simulink model "kestane"  (R2021b)
settings: Solver=VariableStepAuto  StartTime=0.0  StopTime=70  RelTol=1e-3
values from neighbouring files (symbols this model uses):
  g = vpa(simplify(g),4)    [dynamic.m]
  k = 4e-2    (= 0.04)    [trajectory_computation.m]
undefined symbols (not defined in the file or in its folder): sigbuilder_block, X, Y, Z
libraries: sm_lib x139, nesl_utility x13, Contact_Forces_Lib x1
(part 5 of 5)

== system kestane/Kestane/Top spike6 ==
  Brick Solid5 : sm_lib/Body Elements/Brick Solid  GraphicAmbientColor=[0.15 0.15 0.15 1.0]  BasedOnType=Density  BrickDimensions=[k 0.005 0.005]  BrickDimensionUnits=m  CenterOfMass=[0 0 0]  CenterOfMassUnits=cm  GraphicDiffuseColor=[0.5 0.5 0.5]  Density=100  DensityUnits=g/cm^3  DoExposeReferenceFrame=on  GraphicEmissiveColor=[0.0 0.0 0.0 1.0]  ExportEntireGeometry=on  SerializedFrames=<Frames><Frame><Id>Frame1</Id><Value><Name>F1</Name><Origin><Source>GeometricFeature</Source><FeatureName>+x surface</FeatureName></Origin><PrimaryAxis><DefinedDirection>+Z</DefinedDirection><Source>GeometricFeature</Source><SourceDirection>+Z</SourceDirection><FeatureName>+x surface</FeatureName></PrimaryAxis><SecondaryAxis><DefinedDirection>-Y</DefinedDirection><Source>GeometricFeature</Source><SourceDirection>+X</SourceDirection><FeatureName>+x -y curve</FeatureName></SecondaryAxis></Value></Frame><Frame><Id>Frame2</Id><Value><Name>F2</Name><Origin><Source>GeometricFeature</Source><FeatureName>-x surface</FeatureName></Origin><PrimaryAxis><DefinedDirection>-Z</DefinedDirection><Source>GeometricFeature</Source><SourceDirection>+Z</SourceDirection><FeatureName>-x surface</FeatureName></PrimaryAxis><SecondaryAxis><DefinedDirection>-X</DefinedDirection><Source>GeometricFeature</Source><SourceDirection>+X</SourceDirection><FeatureName>+z -x curve</FeatureName></SecondaryAxis></Value></Frame></Frames>  MarkerShape=Sphere  MarkerSize=10  GraphicType=FromGeometry  InertiaType=Custom  Mass=10  MassUnits=g  MomentsOfInertia=[1e-15 1e-15 1e-15]  MomentsOfInertiaUnits=g*cm^2  GraphicOpacity=1.0  ProductsOfInertia=[0 0 0]  ProductsOfInertiaUnits=kg*m^2  GraphicShininess=75  GraphicSpecularColor=[0.5 0.5 0.5 1.0]  GraphicVisPropType=SimpleVisualProperties
  Cylindrical Solid : sm_lib/Body Elements/Cylindrical Solid  GraphicAmbientColor=[0.15 0.15 0.15 1.0]  BasedOnType=Density  CenterOfMass=[0 0 0]  CenterOfMassUnits=cm  GraphicDiffuseColor=[0.5 0.5 0.5]  CylinderLength=r  CylinderLengthUnits=m  CylinderRadius=0.25  CylinderRadiusUnits=cm  Density=100  DensityUnits=g/cm^3  DoExposeReferenceFrame=on  GraphicEmissiveColor=[0.0 0.0 0.0 1.0]  ExportEntireGeometry=on  SerializedFrames=<Frames><Frame><Id>Frame1</Id><Value><Name>F1</Name><Origin><Source>GeometricFeature</Source><FeatureName>top surface</FeatureName></Origin><PrimaryAxis><DefinedDirection>+Z</DefinedDirection><Source>ReferenceFrame</Source><SourceDirection>+Z</SourceDirection><FeatureName></FeatureName></PrimaryAxis><SecondaryAxis><DefinedDirection>+X</DefinedDirection><Source>ReferenceFrame</Source><SourceDirection>+X</SourceDirection><FeatureName></FeatureName></SecondaryAxis></Value></Frame><Frame><Id>Frame2</Id><Value><Name>F2</Name><Origin><Source>GeometricFeature</Source><FeatureName>top surface</FeatureName></Origin><PrimaryAxis><DefinedDirection>+Z</DefinedDirection><Source>ReferenceFrame</Source><SourceDirection>+Z</SourceDirection><FeatureName></FeatureName></PrimaryAxis><SecondaryAxis><DefinedDirection>+X</DefinedDirection><Source>ReferenceFrame</Source><SourceDirection>+X</SourceDirection><FeatureName></FeatureName></SecondaryAxis></Value></Frame></Frames>  MarkerShape=Sphere  MarkerSize=10  GraphicType=FromGeometry  InertiaType=Custom  Mass=50  MassUnits=g  MomentsOfInertia=[1e-15 1e-15 1e-15]  MomentsOfInertiaUnits=g*cm^2  GraphicOpacity=1.0  ProductsOfInertia=[0 0 0]  ProductsOfInertiaUnits=kg*m^2  GraphicShininess=75  GraphicSpecularColor=[0.5 0.5 0.5 1.0]  GraphicVisPropType=SimpleVisualProperties
  Prismatic Joint5 : sm_lib/Joints/Prismatic Joint  JointMode=Normal  SenseConstraintForce=off  SenseConstraintForceX=off  SenseConstraintForceY=off  SenseConstraintForceZ=off  SenseConstraintTorque=off  SenseConstraintTorqueX=off  SenseConstraintTorqueY=off  SenseConstraintTorqueZ=off  SenseTotalForce=off  SenseTotalForceX=off  SenseTotalForceY=off  SenseTotalForceZ=off  SenseTotalTorque=off  SenseTotalTorqueX=off  SenseTotalTorqueY=off  SenseTotalTorqueZ=off  CompositeWrenchDir=FollowerOnBase  CompositeWrenchFrame=BaseFrame  EquilibriumPosition=0  EquilibriumPositionUnits=cm  SpringStiffness=10  SpringStiffnessUnits=N/m  DampingCoefficient=10  DampingCoefficientUnits=N/(m/s)  TorqueActuationMode=NoTorque  MotionActuationMode=ComputedMotion  SensePosition=off  SenseVelocity=off  SenseAcceleration=off  SenseTorqueForce=off  SenseLowerLimitTorqueForce=off  SenseUpperLimitTorqueForce=off  LowerLimitSpecify=on  LowerLimitBound=1  LowerLimitBoundUnits=cm  LowerLimitStiffness=1e3  LowerLimitStiffnessUnits=N/m  LowerLimitDamping=1e3  LowerLimitDampingUnits=N/(m/s)  LowerLimitTransitionRegionWidth=1e-4  LowerLimitTransitionRegionWidthUnits=m  UpperLimitSpecify=on  UpperLimitBound=2  UpperLimitBoundUnits=cm  UpperLimitStiffness=1e4  UpperLimitStiffnessUnits=N/m  UpperLimitDamping=1e4  UpperLimitDampingUnits=N/(m/s)  UpperLimitTransitionRegionWidth=1e-4  UpperLimitTransitionRegionWidthUnits=m  PositionTargetSpecify=on  PositionTargetPriority=High  PositionTargetValue=1.5  PositionTargetValueUnits=cm  VelocityTargetSpecify=on  VelocityTargetPriority=High  VelocityTargetValue=0  VelocityTargetValueUnits=m/s
  Revolute Joint11 : sm_lib/Joints/Revolute Joint  JointMode=Normal  SenseConstraintForce=off  SenseConstraintForceX=off  SenseConstraintForceY=off  SenseConstraintForceZ=off  SenseConstraintTorque=off  SenseConstraintTorqueX=off  SenseConstraintTorqueY=off  SenseConstraintTorqueZ=off  SenseTotalForce=off  SenseTotalForceX=off  SenseTotalForceY=off  SenseTotalForceZ=off  SenseTotalTorque=off  SenseTotalTorqueX=off  SenseTotalTorqueY=off  SenseTotalTorqueZ=off  CompositeWrenchDir=FollowerOnBase  CompositeWrenchFrame=BaseFrame  EquilibriumPosition=0  EquilibriumPositionUnits=deg  SpringStiffness=0  SpringStiffnessUnits=N*m/deg  DampingCoefficient=1e10  DampingCoefficientUnits=N*m/(deg/s)  TorqueActuationMode=NoTorque  MotionActuationMode=ComputedMotion  SensePosition=off  SenseVelocity=off  SenseAcceleration=off  SenseTorqueForce=off  SenseLowerLimitTorqueForce=off  SenseUpperLimitTorqueForce=off  LowerLimitSpecify=on  LowerLimitBound=82  LowerLimitBoundUnits=deg  LowerLimitStiffness=0  LowerLimitStiffnessUnits=N*m/deg  LowerLimitDamping=1e10  LowerLimitDampingUnits=N*m/(deg/s)  LowerLimitTransitionRegionWidth=0.1  LowerLimitTransitionRegionWidthUnits=deg  UpperLimitSpecify=on  UpperLimitBound=98  UpperLimitBoundUnits=deg  UpperLimitStiffness=0  UpperLimitStiffnessUnits=N*m/deg  UpperLimitDamping=1e10  UpperLimitDampingUnits=N*m/(deg/s)  UpperLimitTransitionRegionWidth=0.1  UpperLimitTransitionRegionWidthUnits=deg  PositionTargetSpecify=on  PositionTargetPriority=High  PositionTargetValue=90  PositionTargetValueUnits=deg  VelocityTargetSpecify=off  VelocityTargetPriority=High  VelocityTargetValue=0  VelocityTargetValueUnits=deg/s
  Revolute Joint5 : sm_lib/Joints/Revolute Joint  JointMode=Normal  SenseConstraintForce=off  SenseConstraintForceX=off  SenseConstraintForceY=off  SenseConstraintForceZ=off  SenseConstraintTorque=off  SenseConstraintTorqueX=off  SenseConstraintTorqueY=off  SenseConstraintTorqueZ=off  SenseTotalForce=off  SenseTotalForceX=off  SenseTotalForceY=off  SenseTotalForceZ=off  SenseTotalTorque=off  SenseTotalTorqueX=off  SenseTotalTorqueY=off  SenseTotalTorqueZ=off  CompositeWrenchDir=FollowerOnBase  CompositeWrenchFrame=BaseFrame  EquilibriumPosition=-30  EquilibriumPositionUnits=deg  SpringStiffness=1  SpringStiffnessUnits=N*m/deg  DampingCoefficient=1  DampingCoefficientUnits=N*m/(deg/s)  TorqueActuationMode=NoTorque  MotionActuationMode=ComputedMotion  SensePosition=off  SenseVelocity=off  SenseAcceleration=off  SenseTorqueForce=off  SenseLowerLimitTorqueForce=off  SenseUpperLimitTorqueForce=off  LowerLimitSpecify=on  LowerLimitBound=-31  LowerLimitBoundUnits=deg  LowerLimitStiffness=1e4  LowerLimitStiffnessUnits=N*m/deg  LowerLimitDamping=10  LowerLimitDampingUnits=N*m/(deg/s)  LowerLimitTransitionRegionWidth=0.1  LowerLimitTransitionRegionWidthUnits=deg  UpperLimitSpecify=on  UpperLimitBound=-29  UpperLimitBoundUnits=deg  UpperLimitStiffness=1e4  UpperLimitStiffnessUnits=N*m/deg  UpperLimitDamping=10  UpperLimitDampingUnits=N*m/(deg/s)  UpperLimitTransitionRegionWidth=0.1  UpperLimitTransitionRegionWidthUnits=deg  PositionTargetSpecify=on  PositionTargetPriority=High  PositionTargetValue=-30  PositionTargetValueUnits=deg  VelocityTargetSpecify=on  VelocityTargetPriority=High  VelocityTargetValue=0  VelocityTargetValueUnits=deg/s
  Rigid Transform10 : sm_lib/Frames and Transforms/Rigid Transform  TranslationMethod=None  TranslationStandardOffset=0  TranslationLengthUnit=m  TranslationStandardAxis=+Z  TranslationCartesianOffset=[0 0 0]  TranslationROffset=0  TranslationROffsetUnits=m  TranslationZOffset=0  TranslationZOffsetUnits=m  TranslationThetaOffset=0  TranslationThetaOffsetUnits=deg  RotationMethod=StandardAxis  RotationAngleUnits=deg  RotationStandardAxis=+X  RotationAngle=90.0  RotationArbitraryAxis=[0 0 1]  FollAlignAxisA=+X  BaseAlignAxisA=+Y  FollAlignAxisB=+Y  BaseAlignAxisB=+Z  RotationSequenceAxes=FollowerAxes  RotationSequence=XYX  RotationSequenceAngles=[0 0 0]  RotationSequenceAnglesUnits=deg  RotationMatrix=[1 0 0; 0 1 0; 0 0 1]
  Rigid Transform16 : sm_lib/Frames and Transforms/Rigid Transform  TranslationMethod=StandardAxis  TranslationStandardOffset=0.5  TranslationLengthUnit=cm  TranslationStandardAxis=+Z  TranslationCartesianOffset=[0 0 0]  TranslationROffset=0  TranslationROffsetUnits=m  TranslationZOffset=0  TranslationZOffsetUnits=m  TranslationThetaOffset=0  TranslationThetaOffsetUnits=deg  RotationMethod=None  RotationAngleUnits=deg  RotationStandardAxis=+Z  RotationAngle=0.0  RotationArbitraryAxis=[0 0 1]  FollAlignAxisA=+X  BaseAlignAxisA=+Y  FollAlignAxisB=+Y  BaseAlignAxisB=+Z  RotationSequenceAxes=FollowerAxes  RotationSequence=XYX  RotationSequenceAngles=[0 0 0]  RotationSequenceAnglesUnits=deg  RotationMatrix=[1 0 0; 0 1 0; 0 0 1]
  Rigid Transform22 : sm_lib/Frames and Transforms/Rigid Transform  TranslationMethod=None  TranslationStandardOffset=0  TranslationLengthUnit=m  TranslationStandardAxis=+Z  TranslationCartesianOffset=[0 0 0]  TranslationROffset=0  TranslationROffsetUnits=m  TranslationZOffset=0  TranslationZOffsetUnits=m  TranslationThetaOffset=0  TranslationThetaOffsetUnits=deg  RotationMethod=StandardAxis  RotationAngleUnits=deg  RotationStandardAxis=+X  RotationAngle=90.0  RotationArbitraryAxis=[0 0 1]  FollAlignAxisA=+X  BaseAlignAxisA=+Y  FollAlignAxisB=+Y  BaseAlignAxisB=+Z  RotationSequenceAxes=FollowerAxes  RotationSequence=XYX  RotationSequenceAngles=[0 0 0]  RotationSequenceAnglesUnits=deg  RotationMatrix=[1 0 0; 0 1 0; 0 0 1]
  Rigid Transform5 : sm_lib/Frames and Transforms/Rigid Transform  TranslationMethod=Cartesian  TranslationStandardOffset=0  TranslationLengthUnit=cm  TranslationStandardAxis=+Z  TranslationCartesianOffset=[-1.5*sqrt(3) 0 +1.5]  TranslationROffset=0  TranslationROffsetUnits=m  TranslationZOffset=0  TranslationZOffsetUnits=m  TranslationThetaOffset=0  TranslationThetaOffsetUnits=deg  RotationMethod=RotationMatrix  RotationAngleUnits=deg  RotationStandardAxis=+Z  RotationAngle=0.0  RotationArbitraryAxis=[0 0 1]  FollAlignAxisA=+X  BaseAlignAxisA=+Y  FollAlignAxisB=+Y  BaseAlignAxisB=+Z  RotationSequenceAxes=FollowerAxes  RotationSequence=XYX  RotationSequenceAngles=[0 0 0]  RotationSequenceAnglesUnits=deg  RotationMatrix=[-1 0 0;0 0 -1; 0 -1 0]
  Spatial Contact Force5 : sm_lib/Forces and Torques/Spatial Contact Force  CoefficientOfDynamicFriction=0.5  CoefficientOfStaticFriction=0.7  SenseContactBaseRotation=off  SenseContactBaseTranslation=off  NormalDamping=10  NormalDampingUnits=N/(m/s)  SenseContactFollowerRotation=off  SenseContactFollowerTranslation=off  SenseContactSignal=off  NormalStiffness=1e6  NormalStiffnessUnits=N/m  FrictionalCriticalVelocity=1e-3  FrictionalCriticalVelocityUnits=m/s  ZeroCrossDetectContactStartAndEnd=off  FrictionType=SmoothStickSlip  SenseFrictionalForceMagnitude=off  SenseNormalForceMagnitude=off  NormalForceType=SmoothSpringDamper  SenseNormalVelocity=off  SenseSeparationDistance=off  SenseTangentialVelocity=off  SenseTangentialVelocityMagnitude=off  NormalTransitionRegionWidth=1e-4  NormalTransitionRegionWidthUnits=m
  Spherical Solid5 : sm_lib/Body Elements/Spherical Solid  GraphicAmbientColor=[0.15 0.15 0.15 1.0]  BasedOnType=Mass  CenterOfMass=[0 0 0]  CenterOfMassUnits=m  GraphicDiffuseColor=[0.5 0.5 0.5]  Density=1000  DensityUnits=kg/m^3  DoExposeReferenceFrame=on  GraphicEmissiveColor=[0.0 0.0 0.0 1.0]  ExportEntireGeometry=on  SerializedExposedGeometries=<ExposedGeometries><ExposedGeometry><RawGeometryId>entire</RawGeometryId><ExposedGeometryId>G</ExposedGeometryId></ExposedGeometry></ExposedGeometries>  SerializedFrames=<Frames/>  MarkerShape=Sphere  MarkerSize=10  GraphicType=FromGeometry  InertiaType=CalculateFromGeometry  Mass=5  MassUnits=g  MomentsOfInertia=[1 1 1]  MomentsOfInertiaUnits=kg*m^2  GraphicOpacity=1.0  ProductsOfInertia=[0 0 0]  ProductsOfInertiaUnits=kg*m^2  GraphicShininess=75  GraphicSpecularColor=[0.5 0.5 0.5 1.0]  SphereRadius=0.5  SphereRadiusUnits=cm  GraphicVisPropType=SimpleVisualProperties
  Conn1 : PMIOPort  Side=Left
  Conn5 : PMIOPort  Port=2  Side=Left
  connections:
  Prismatic Joint5/LConn1 -- Brick Solid5/LConn1
  Rigid Transform10/RConn1 -- Revolute Joint11/LConn1
  Rigid Transform5/RConn1 -- Revolute Joint5/LConn1
  Rigid Transform10/LConn1 -- Revolute Joint5/RConn1
  Spherical Solid5/LConn1 -- Spatial Contact Force5/RConn1
  Rigid Transform16/RConn1 -- Spherical Solid5/RConn1
  Prismatic Joint5/RConn1 -- Cylindrical Solid/LConn2
  Rigid Transform22/LConn1 -- Revolute Joint11/RConn1
  Cylindrical Solid/LConn1 -- Rigid Transform16/LConn1
  Rigid Transform22/RConn1 -- Brick Solid5/LConn2
  Spatial Contact Force5/LConn1 -- Conn5/RConn1
  Conn1/RConn1 -- Rigid Transform5/LConn1

== system kestane/Kestane/Spike 1/Signal Builder ==
  Demux : Demux  Tag=STV Demux  Outputs=3
      settings: DisplayOption=none
  FromWs : FromWorkspace  Tag=STV FromWs  VariableName=tuvar
      SigBuilderData=|
      | common.afterFinalStr = 'Extrapolate'
      | common.sampleTime = 0
      | dataSet.timeRange = [0 70]
      | dataSet.name = 'Group 1'
      | sbobj.Groups.Name = 'Group 1'
      | sbobj.Groups.Signals(1).Name = 'theta1v'
      | sbobj.Groups.Signals(1).XData = [0 1 1.02004008016 1.04008016032 1.06012024048 1.08016032064 1.1002004008 1.12024048096 1.14028056112 1.16032064128 1.18036072144 1.2004008016 ... (5001 elements, 1x5001)]
      | sbobj.Groups.Signals(1).YData = [-1.33121558998e-05 -1.33121558998e-05 -5.28852062004e-05 -0.000170609462846 -0.000364414136278 -0.00063215837707 -0.000971723764753 -0.00138101533953 -0.00185796251377 -0.00240051986857 -0.00300666784074 -0.00367441330488 ... (5001 elements, 1x5001)]
      | sbobj.Groups.Signals(2).Name = 'theta2v'
      | sbobj.Groups.Signals(2).XData = [0 1 1.02004008016 1.04008016032 1.06012024048 1.08016032064 1.1002004008 1.12024048096 1.14028056112 1.16032064128 1.18036072144 1.2004008016 ... (5002 elements, 1x5002)]
      | sbobj.Groups.Signals(2).YData = [9.17654507937e-07 9.17654507937e-07 3.66528587481e-06 1.18935666149e-05 2.5572133272e-05 4.46698421197e-05 6.91564068234e-05 9.90026718162e-05 0.000134180855199 0.000174664762492 0.000220429972497 0.000271453996453 ... (5002 elements, 1x5002)]
      | sbobj.Groups.Signals(3).Name = 'd3v'
      | sbobj.Groups.Signals(3).XData = [0 1 1.02004008016 1.04008016032 1.06012024048 1.08016032064 1.1002004008 1.12024048096 1.14028056112 1.16032064128 1.18036072144 1.2004008016 ... (5002 elements, 1x5002)]
      | sbobj.Groups.Signals(3).YData = [-2.27265007507e-07 -2.27265007507e-07 -9.03146913159e-07 -2.91455572836e-06 -6.22754426326e-06 -1.08066210217e-05 -1.66160796084e-05 -2.36198607756e-05 -3.17814304776e-05 -4.10636731864e-05 -5.14287997626e-05 -6.28382692144e-05 ... (5002 elements, 1x5002)]
      | sbobj.Groups.TimeRange = [0 70]
  theta1v : Outport  Tag=STV Outport
  theta2v : Outport  Tag=STV Outport  Port=2
  d3v : Outport  Tag=STV Outport  Port=3
  wires:
  Demux/1 -> theta1v/1
  FromWs/1 -> Demux/1
  Demux/2 -> theta2v/1
  Demux/3 -> d3v/1

== system kestane/Kestane/Spike 4/Spike 1 Driver ==
  Demux : Demux  Tag=STV Demux  Outputs=3
      settings: DisplayOption=none
  FromWs : FromWorkspace  Tag=STV FromWs  VariableName=tuvar
      SigBuilderData=|
      | common.afterFinalStr = 'Extrapolate'
      | common.sampleTime = 0
      | dataSet.timeRange = [0 70]
      | dataSet.name = 'Group 1'
      | sbobj.Groups.Name = 'Group 1'
      | sbobj.Groups.Signals(1).Name = 'theta1'
      | sbobj.Groups.Signals(1).XData = [0 1 1.02004008016 1.04008016032 1.06012024048 1.08016032064 1.1002004008 1.12024048096 1.14028056112 1.16032064128 1.18036072144 1.2004008016 ... (4997 elements, 1x4997)]
      | sbobj.Groups.Signals(1).YData = [0.523598775598 0.523598775598 0.523598509355 0.52359666019 0.523591684977 0.523582083625 0.523566398642 0.523543214674 0.523511158028 0.523468896173 0.523415137233 0.52334862946 ... (4997 elements, 1x4997)]
      | sbobj.Groups.Signals(2).Name = 'd3'
      | sbobj.Groups.Signals(2).XData = [0 1 1.02004008016 1.04008016032 1.06012024048 1.08016032064 1.1002004008 1.12024048096 1.14028056112 1.16032064128 1.18036072144 1.2004008016 ... (4998 elements, 1x4998)]
      | sbobj.Groups.Signals(2).YData = [0.0120221607105 0.0120221607105 0.0120221561652 0.0120221245847 0.012022039583 0.0120218754829 0.0120216073182 0.0120212108397 0.0120206625237 0.0120199395825 0.0120190199768 0.0120178824305 ... (4998 elements, 1x4998)]
      | sbobj.Groups.Signals(3).Name = 'theta2'
      | sbobj.Groups.Signals(3).XData = [0 1 1.02004008016 1.04008016032 1.06012024048 1.08016032064 1.1002004008 1.12024048096 1.14028056112 1.16032064128 1.18036072144 1.2004008016 ... (4998 elements, 1x4998)]
      | sbobj.Groups.Signals(3).YData = [1.7345311581 1.7345311581 1.73453113975 1.73453101149 1.73453066401 1.73452998861 1.73452887721 1.73452722235 1.73452491711 1.73452185512 1.73451793052 1.73451303792 ... (4998 elements, 1x4998)]
      | sbobj.Groups.TimeRange = [0 70]
  theta1 : Outport  Tag=STV Outport
  d3 : Outport  Tag=STV Outport  Port=2
  theta2 : Outport  Tag=STV Outport  Port=3
  wires:
  FromWs/1 -> Demux/1
  Demux/1 -> theta1/1
  Demux/2 -> d3/1
  Demux/3 -> theta2/1

== matlab function kestane/Kestane/Spike 1/MATLAB Function ==
  data: theta1 input; t1 output; theta2 input; d3 input; theta1v input; theta2v input; d3v input; theta1vd input; theta2vd input; d3vd input; theta1d input; theta2d input; d3d input; t2 output; t3 output
function [t1,t2,t3] = force_control(theta1,theta2,d3,theta1v,theta2v,d3v,theta1vd,theta2vd,d3vd,theta1d,theta2d,d3d)
x = (0.04+d3);
J = [-x*sin(theta1)*sin(theta2) x*cos(theta1)*cos(theta2) cos(theta1)*sin(theta2);
    x*cos(theta1)*sin(theta2) x*sin(theta1)*cos(theta2) sin(theta1)*sin(theta2);
    0 x*sin(theta2) -cos(theta2)];
K = [1e4 0 0;0 1e4 0;0 0 1e4];
L = [1e2 0 0;0 0 0;0 0 1e2];
error = [-(theta1-theta1d);-(theta2-theta2d);-(d3 -d3d)];
errorv = [theta1vd-theta1v;theta2vd-theta2v;d3vd-d3v];
t = J'*K*J*error + L*errorv;
% external = J'*[0;-nforce;0];
t1 = t(1); %+ external(1);
t2 = t(2); %+ external(2);
t3 = t(3); %+ external(3);                                                 
end
